simulink model "Estimationdataset1"  (R2023b)
settings: Solver=FixedStepAuto  StartTime=0.0  StopTime=60  FixedStep=1/4096  RelTol=1e-3
(part 1 of 2)
settings Model: Creator=ashle  LastModifiedBy=ashle

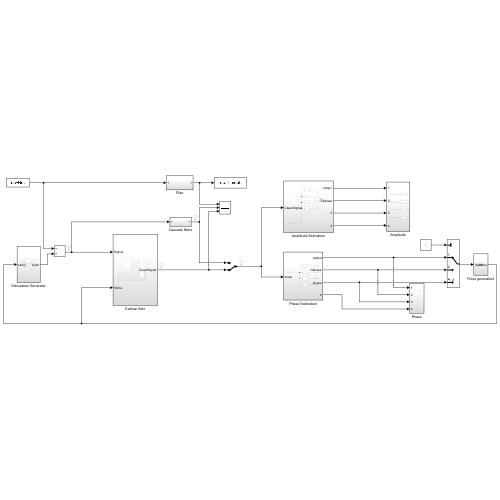
[thumbnail: Simulink's stored preview of the top-level diagram]
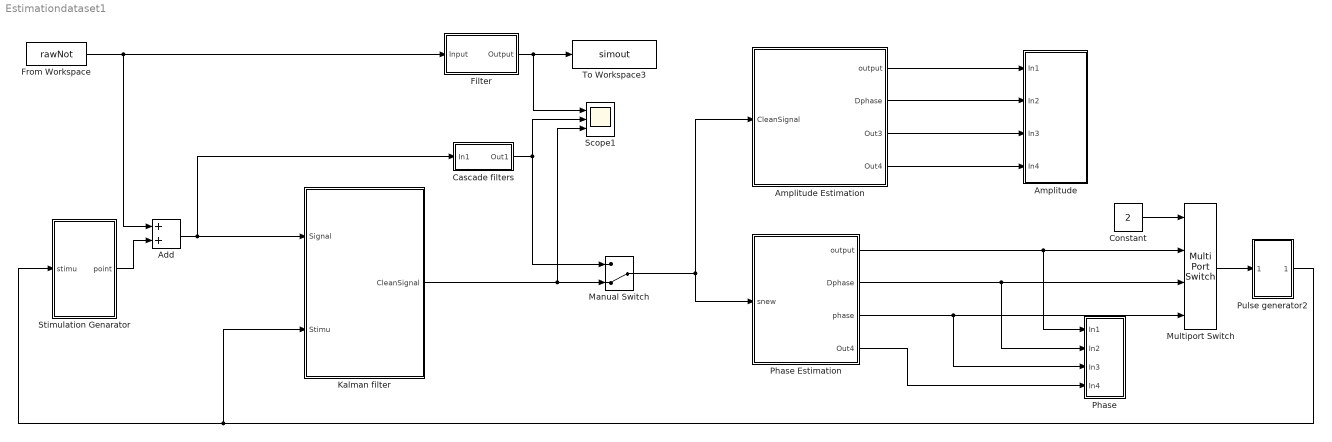
== system Estimationdataset1 ==
  Add : Sum
  Amplitude : Subsystem
  Amplitude Estimation : Subsystem
  Cascade filters : Subsystem
  Constant : Constant  Value=2
  Filter : Subsystem  Tag=FilterWizardSubSystem
      settings: ErrorFcn=dspFilterRealizedInBasicElemsAlgLoopErrFcnCallback
  From Workspace : FromWorkspace  VariableName=rawNot  SampleTime=1/4096
  Kalman filter : Subsystem
  Manual Switch : ManualSwitch  CurrentSetting=0
  Multiport Switch : MultiPortSwitch  SaturateOnIntegerOverflow=off  InputSameDT=off
  Phase : Subsystem
  Phase Estimation : Subsystem
  Pulse generator2 : Subsystem
  Scope1 : Scope  NumInputPorts=3
  Stimulation Genarator : Subsystem
  To Workspace3 : ToWorkspace  VariableName=simout  SampleTime=-1
      settings: Save2DSignal=2-D array (concatenate along first dimension)
  wires:
  Add/1 -> Cascade filters/1(In1), Kalman filter/1(Signal)
  From Workspace/1 -> Filter/1(Input), Add/1
  Stimulation Genarator/1(point) -> Add/2
  Constant/1 -> Multiport Switch/1
  Cascade filters/1(Out1) -> Scope1/2, Manual Switch/1
  Filter/1(Output) -> Scope1/1, To Workspace3/1
  Multiport Switch/1 -> Pulse generator2/1(input)
  Pulse generator2/1(Stimu) -> Stimulation Genarator/1(stimu), Kalman filter/2(Stimu)
  Manual Switch/1 -> Phase Estimation/1(snew), Amplitude Estimation/1(CleanSignal)
  Amplitude Estimation/1(output) -> Amplitude/1(In1)
  Amplitude Estimation/2(Dphase) -> Amplitude/2(In2)
  Amplitude Estimation/3(Out3) -> Amplitude/3(In3)
  Amplitude Estimation/4(Out4) -> Amplitude/4(In4)
  Phase Estimation/1(output) -> Phase/1(In1), Multiport Switch/2
  Phase Estimation/2(Dphase) -> Phase/2(In2), Multiport Switch/3
  Phase Estimation/3(phase) -> Phase/3(In3), Multiport Switch/4
  Phase Estimation/4(Out4) -> Phase/4(In4)
  Kalman filter/1(CleanSignal) -> Scope1/3, Manual Switch/2

== system Estimationdataset1/Amplitude ==
  In1 : Inport
  In2 : Inport  Port=2
  In3 : Inport  Port=3
  In4 : Inport  Port=4
  MW : ToWorkspace  VariableName=simout7  SampleTime=-1
      settings: Save2DSignal=2-D array (concatenate along first dimension)
  NRO : ToWorkspace  VariableName=simout5  SampleTime=-1
      settings: Save2DSignal=2-D array (concatenate along first dimension)
  SS : ToWorkspace  VariableName=simout8  SampleTime=-1
      settings: Save2DSignal=2-D array (concatenate along first dimension)
  ecHT : ToWorkspace  VariableName=simout6  SampleTime=-1
      settings: Save2DSignal=2-D array (concatenate along first dimension)
  wires:
  In2/1 -> NRO/1
  In4/1 -> SS/1
  In1/1 -> ecHT/1
  In3/1 -> MW/1

== system Estimationdataset1/Amplitude Estimation ==
  CleanSignal : Inport
  Hilbert+AR1 : Subsystem
  Moving window : Subsystem
  Non-Resonant Filter1 : Subsystem
  State Space1 : Subsystem
  output : Outport
  Dphase : Outport  Port=2
  Out3 : Outport  Port=3
  Out4 : Outport  Port=4
  wires:
  CleanSignal/1 -> Non-Resonant Filter1/1(snew), Hilbert+AR1/1(input), Moving window/1(input), State Space1/1(CleanSignal)
  Hilbert+AR1/1(output) -> output/1
  Moving window/1(Out1) -> Out3/1
  Non-Resonant Filter1/1(Dphase) -> Dphase/1
  State Space1/1(Out2) -> Out4/1

== system Estimationdataset1/Cascade filters ==
  In1 : Inport
  Filter : Subsystem  Tag=FilterWizardSubSystem
      settings: ErrorFcn=dspFilterRealizedInBasicElemsAlgLoopErrFcnCallback
  Filter1 : Subsystem  Tag=FilterWizardSubSystem
      settings: ErrorFcn=dspFilterRealizedInBasicElemsAlgLoopErrFcnCallback
  Filter2 : Subsystem  Tag=FilterWizardSubSystem
      settings: ErrorFcn=dspFilterRealizedInBasicElemsAlgLoopErrFcnCallback
  Out1 : Outport
  wires:
  In1/1 -> Filter/1(Input)
  Filter/1(Output) -> Filter1/1(Input)
  Filter1/1(Output) -> Filter2/1(Input)
  Filter2/1(Output) -> Out1/1

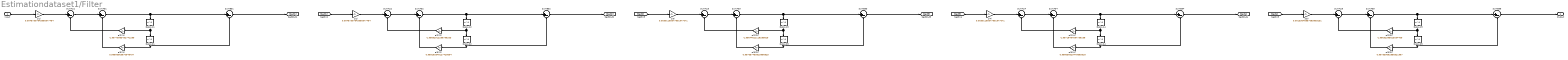
== system Estimationdataset1/Filter ==
  Input : Inport
  Delay{11..15,21..25} (10 alike) : Delay  DelayLength=1  InitialCondition=0
  SumA{21..25,31..35} (10 alike) : Sum  Inputs=|+-  RndMeth=Nearest  SaturateOnIntegerOverflow=on  OutDataTypeStr=Inherit: Same as first input
  SumB{31..35} (5 alike) : Sum  Inputs=|+-  RndMeth=Nearest  SaturateOnIntegerOverflow=on  OutDataTypeStr=Inherit: Same as first input
  a(2)(1) : Gain  Gain=-1.99770983432741289  ParamDataTypeStr=double  RndMeth=Nearest  SaturateOnIntegerOverflow=on  OutDataTypeStr=Inherit: Same as input
  a(2)(2) : Gain  Gain=-1.99852912286796203  ParamDataTypeStr=double  RndMeth=Nearest  SaturateOnIntegerOverflow=on  OutDataTypeStr=Inherit: Same as input
  a(2)(3) : Gain  Gain=-1.99644621118280829  ParamDataTypeStr=double  RndMeth=Nearest  SaturateOnIntegerOverflow=on  OutDataTypeStr=Inherit: Same as input
  a(2)(4) : Gain  Gain=-1.99718487687736168  ParamDataTypeStr=double  RndMeth=Nearest  SaturateOnIntegerOverflow=on  OutDataTypeStr=Inherit: Same as input
  a(2)(5) : Gain  Gain=-1.99632395623034409  ParamDataTypeStr=double  RndMeth=Nearest  SaturateOnIntegerOverflow=on  OutDataTypeStr=Inherit: Same as input
  a(3)(1) : Gain  Gain=0.99906063670948797  ParamDataTypeStr=double  RndMeth=Nearest  SaturateOnIntegerOverflow=on  OutDataTypeStr=Inherit: Same as input
  a(3)(2) : Gain  Gain=0.999293348127428094  ParamDataTypeStr=double  RndMeth=Nearest  SaturateOnIntegerOverflow=on  OutDataTypeStr=Inherit: Same as input
  a(3)(3) : Gain  Gain=0.997657459515996825  ParamDataTypeStr=double  RndMeth=Nearest  SaturateOnIntegerOverflow=on  OutDataTypeStr=Inherit: Same as input
  a(3)(4) : Gain  Gain=0.998036029478669318  ParamDataTypeStr=double  RndMeth=Nearest  SaturateOnIntegerOverflow=on  OutDataTypeStr=Inherit: Same as input
  a(3)(5) : Gain  Gain=0.997339062858321967  ParamDataTypeStr=double  RndMeth=Nearest  SaturateOnIntegerOverflow=on  OutDataTypeStr=Inherit: Same as input
  s(1) : Gain  Gain=0.00457307843590577454  ParamDataTypeStr=double  RndMeth=Nearest  SaturateOnIntegerOverflow=on  OutDataTypeStr=Inherit: Same as input
  s(2) : Gain  Gain=0.00457307843590577454  ParamDataTypeStr=double  RndMeth=Nearest  SaturateOnIntegerOverflow=on  OutDataTypeStr=Inherit: Same as input
  s(3) : Gain  Gain=0.00301199377801977071  ParamDataTypeStr=double  RndMeth=Nearest  SaturateOnIntegerOverflow=on  OutDataTypeStr=Inherit: Same as input
  s(4) : Gain  Gain=0.00301199377801977071  ParamDataTypeStr=double  RndMeth=Nearest  SaturateOnIntegerOverflow=on  OutDataTypeStr=Inherit: Same as input
  s(5) : Gain  Gain=0.00133046857083903231  ParamDataTypeStr=double  RndMeth=Nearest  SaturateOnIntegerOverflow=on  OutDataTypeStr=Inherit: Same as input
  Output : Outport
  wires:
  Input/1 -> s(1)/1
  s(1)/1 -> SumA21/1
  SumA21/1 -> SumA31/1
  SumA31/1 -> SumB31/1, Delay11/1
  SumB31/1 -> [Sect1]
  a(2)(1)/1 -> SumA21/2
  Delay11/1 -> a(2)(1)/1, Delay21/1
  a(3)(1)/1 -> SumA31/2
  Delay21/1 -> a(3)(1)/1, SumB31/2
  [Sect1] -> s(2)/1
  s(2)/1 -> SumA22/1
  SumA22/1 -> SumA32/1
  SumA32/1 -> SumB32/1, Delay12/1
  SumB32/1 -> [Sect2]
  a(2)(2)/1 -> SumA22/2
  Delay12/1 -> a(2)(2)/1, Delay22/1
  a(3)(2)/1 -> SumA32/2
  Delay22/1 -> a(3)(2)/1, SumB32/2
  [Sect2] -> s(3)/1
  s(3)/1 -> SumA23/1
  SumA23/1 -> SumA33/1
  SumA33/1 -> SumB33/1, Delay13/1
  SumB33/1 -> [Sect3]
  a(2)(3)/1 -> SumA23/2
  Delay13/1 -> a(2)(3)/1, Delay23/1
  a(3)(3)/1 -> SumA33/2
  Delay23/1 -> a(3)(3)/1, SumB33/2
  [Sect3] -> s(4)/1
  s(4)/1 -> SumA24/1
  SumA24/1 -> SumA34/1
  SumA34/1 -> SumB34/1, Delay14/1
  SumB34/1 -> [Sect4]
  a(2)(4)/1 -> SumA24/2
  Delay14/1 -> a(2)(4)/1, Delay24/1
  a(3)(4)/1 -> SumA34/2
  Delay24/1 -> a(3)(4)/1, SumB34/2
  [Sect4] -> s(5)/1
  s(5)/1 -> SumA25/1
  SumA25/1 -> SumA35/1
  SumA35/1 -> SumB35/1, Delay15/1
  SumB35/1 -> Output/1
  a(2)(5)/1 -> SumA25/2
  Delay15/1 -> a(2)(5)/1, Delay25/1
  a(3)(5)/1 -> SumA35/2
  Delay25/1 -> a(3)(5)/1, SumB35/2

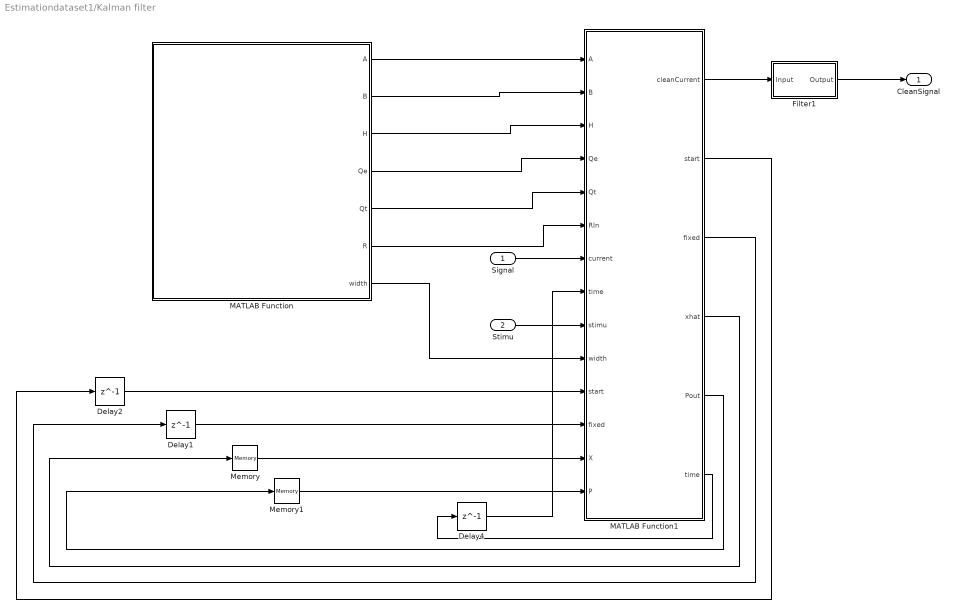
== system Estimationdataset1/Kalman filter ==
  Signal : Inport
  Stimu : Inport  Port=2
  Delay1 : Delay  DelayLength=1  InitialCondition=0
  Delay2 : Delay  DelayLength=1  InitialCondition=0
  Delay4 : Delay  DelayLength=1  InitialCondition=0
  Filter1 : Subsystem  Tag=FilterWizardSubSystem
      settings: ErrorFcn=dspFilterRealizedInBasicElemsAlgLoopErrFcnCallback
  MATLAB Function : MATLAB Function  TreatAsAtomicUnit=on
  MATLAB Function1 : MATLAB Function  TreatAsAtomicUnit=on
  Memory : Memory  InheritSampleTime=on
  Memory1 : Memory  InheritSampleTime=on
  CleanSignal : Outport
  wires:
  Stimu/1 -> MATLAB Function1/9(stimu)
  Memory1/1 -> MATLAB Function1/14(P)
  MATLAB Function1/3(fixed) -> Delay1/1
  Delay1/1 -> MATLAB Function1/12("fixed ")
  MATLAB Function1/2(start) -> Delay2/1
  Delay2/1 -> MATLAB Function1/11("start ")
  Memory/1 -> MATLAB Function1/13(X)
  MATLAB Function1/4(xhat) -> Memory/1
  MATLAB Function1/5(Pout) -> Memory1/1
  MATLAB Function/1(A) -> MATLAB Function1/1(A)
  MATLAB Function/2(B) -> MATLAB Function1/2(B)
  MATLAB Function/3(H) -> MATLAB Function1/3(H)
  MATLAB Function/4(Qe) -> MATLAB Function1/4(Qe)
  MATLAB Function/5(Qt) -> MATLAB Function1/5(Qt)
  MATLAB Function/6(R) -> MATLAB Function1/6(RIn)
  MATLAB Function1/1(cleanCurrent) -> Filter1/1(Input)
  MATLAB Function/7(width) -> MATLAB Function1/10(width)
  Signal/1 -> MATLAB Function1/7(current)
  MATLAB Function1/6(time) -> Delay4/1
  Delay4/1 -> MATLAB Function1/8("time ")
  Filter1/1(Output) -> CleanSignal/1

== system Estimationdataset1/Phase ==
  In1 : Inport
  In2 : Inport  Port=2
  In3 : Inport  Port=3
  In4 : Inport  Port=4
  Scope3 : Scope
  To Workspace : ToWorkspace  VariableName=simout2  SampleTime=-1
      settings: Save2DSignal=2-D array (concatenate along first dimension)
  To Workspace1 : ToWorkspace  VariableName=simout1  SampleTime=-1
      settings: Save2DSignal=2-D array (concatenate along first dimension)
  To Workspace2 : ToWorkspace  VariableName=simout3  SampleTime=-1
      settings: Save2DSignal=2-D array (concatenate along first dimension)
  To Workspace4 : ToWorkspace  VariableName=simout4  SampleTime=-1
      settings: Save2DSignal=2-D array (concatenate along first dimension)
  wires:
  In1/1 -> To Workspace1/1
  In4/1 -> To Workspace4/1
  In3/1 -> To Workspace2/1
  In2/1 -> Scope3/1, To Workspace/1

== system Estimationdataset1/Phase Estimation ==
  snew : Inport
  Hilbert+AR : Subsystem
  Non-Resonant Filter : Subsystem
  State Space : Subsystem
  Zero-crossing : Subsystem
  output : Outport
  Dphase : Outport  Port=2
  phase : Outport  Port=3
  Out4 : Outport  Port=4
  wires:
  Non-Resonant Filter/1(Dphase) -> Dphase/1
  Hilbert+AR/1(output) -> output/1
  Zero-crossing/1(phase) -> phase/1
  snew/1 -> Hilbert+AR/1(input), Non-Resonant Filter/1(snew), State Space/1(CleanSignal), Zero-crossing/1(input)
  State Space/1(Out2) -> Out4/1

== system Estimationdataset1/Pulse generator2 ==
  input : Inport
  Delay5 : Delay  DelayLength=1  InitialCondition=0
  MATLAB Function1 : MATLAB Function  TreatAsAtomicUnit=on
  Stimu : Outport
  wires:
  MATLAB Function1/1(out) -> Delay5/1
  Delay5/1 -> MATLAB Function1/2(previous), Stimu/1
  input/1 -> MATLAB Function1/1(input)

== system Estimationdataset1/Stimulation Genarator ==
  stimu : Inport
  Delay4 : Delay  DelayLength=1  InitialCondition=1
  Enabled Subsystem : Subsystem  TreatAsAtomicUnit=on
  MATLAB Function : MATLAB Function  TreatAsAtomicUnit=on
  Memory : Memory  InheritSampleTime=on  LinearizeAsDelay=on
  point : Outport
  wires:
  MATLAB Function/2(index) -> Delay4/1
  Delay4/1 -> MATLAB Function/3("index ")
  Memory/1 -> MATLAB Function/1(stimulation)
  Enabled Subsystem/1(Out1) -> Memory/1
  MATLAB Function/1(point) -> point/1
  stimu/1 -> Enabled Subsystem/Enable, MATLAB Function/2(stimu)

== system Estimationdataset1/Amplitude Estimation/Hilbert+AR1 ==
  input : Inport
  Buffer : Buffer  N=500  V=499  OutputFrames=off
  Hilbert+AR : MATLAB Function  TreatAsAtomicUnit=on
  output : Outport
  wires:
  Hilbert+AR/1(amp) -> output/1
  input/1 -> Buffer/1
  Buffer/1 -> Hilbert+AR/1(input)

== system Estimationdataset1/Amplitude Estimation/Moving window ==
  input : Inport
  Buffer : Buffer  N=800  V=799  OutputFrames=off
  MATLAB Function : MATLAB Function  TreatAsAtomicUnit=on
  Out1 : Outport
  wires:
  input/1 -> Buffer/1
  Buffer/1 -> MATLAB Function/1(input)
  MATLAB Function/1(amp) -> Out1/1

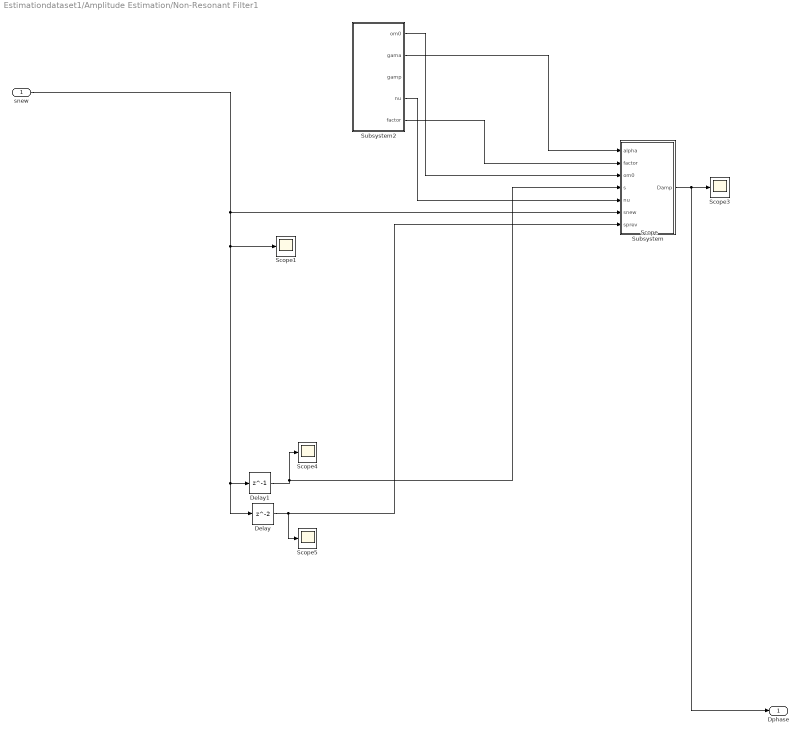
== system Estimationdataset1/Amplitude Estimation/Non-Resonant Filter1 ==
  snew : Inport
  Delay : Delay  InitialCondition=0
  Delay1 : Delay  DelayLength=1  InitialCondition=0
  Scope{,1,3..5} (5 alike) : Scope
  Subsystem : Subsystem
  Subsystem2 : Subsystem
  Dphase : Outport
  wires:
  Delay/1 -> Scope5/1, Subsystem/7(sprev)
  Subsystem2/4(nu) -> Subsystem/5(nu)
  Delay1/1 -> Scope4/1, Subsystem/4(s)
  Subsystem2/1(om0) -> Subsystem/3(om0)
  Subsystem/1(Damp) -> Dphase/1, Scope3/1
  Subsystem2/2(gama) -> Subsystem/1(alpha)
  Subsystem2/5(factor) -> Subsystem/2(factor)
  snew/1 -> Scope1/1, Delay1/1, Delay/1, Subsystem/6(snew)

== system Estimationdataset1/Amplitude Estimation/State Space1 ==
  CleanSignal : Inport
  MATLAB Function2 : MATLAB Function  TreatAsAtomicUnit=on
  MATLAB Function3 : MATLAB Function  TreatAsAtomicUnit=on
  Subsystem : Subsystem
  Out2 : Outport
  wires:
  MATLAB Function2/1(freq) -> MATLAB Function3/1(freq)
  MATLAB Function2/3(ampVec) -> MATLAB Function3/3(ampVector)
  MATLAB Function2/4(sigmaFreqs) -> MATLAB Function3/4(sigmaFreqs)
  MATLAB Function2/2(Fs) -> MATLAB Function3/2(Fs)
  Subsystem/1(Out1) -> Out2/1
  MATLAB Function2/5(sigmaObs) -> Subsystem/1(sigmaObs)
  MATLAB Function3/1(phi) -> Subsystem/2(phi)
  MATLAB Function3/2(Q) -> Subsystem/3(Q)
  MATLAB Function3/3(M) -> Subsystem/4(M)
  CleanSignal/1 -> Subsystem/5(y2)

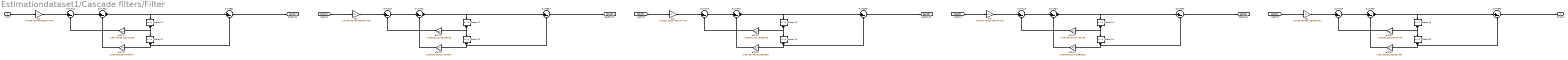
== system Estimationdataset1/Cascade filters/Filter ==
  Input : Inport
  Delay{11..15,21..25} (10 alike) : Delay  DelayLength=1  InitialCondition=0
  SumA{21..25,31..35} (10 alike) : Sum  Inputs=|+-  RndMeth=Nearest  SaturateOnIntegerOverflow=on  OutDataTypeStr=Inherit: Same as first input
  SumB{31..35} (5 alike) : Sum  Inputs=|+-  RndMeth=Nearest  SaturateOnIntegerOverflow=on  OutDataTypeStr=Inherit: Same as first input
  a(2)(1) : Gain  Gain=-1.99770983432741289  ParamDataTypeStr=double  RndMeth=Nearest  SaturateOnIntegerOverflow=on  OutDataTypeStr=Inherit: Same as input
  a(2)(2) : Gain  Gain=-1.99852912286796203  ParamDataTypeStr=double  RndMeth=Nearest  SaturateOnIntegerOverflow=on  OutDataTypeStr=Inherit: Same as input
  a(2)(3) : Gain  Gain=-1.99644621118280829  ParamDataTypeStr=double  RndMeth=Nearest  SaturateOnIntegerOverflow=on  OutDataTypeStr=Inherit: Same as input
  a(2)(4) : Gain  Gain=-1.99718487687736168  ParamDataTypeStr=double  RndMeth=Nearest  SaturateOnIntegerOverflow=on  OutDataTypeStr=Inherit: Same as input
  a(2)(5) : Gain  Gain=-1.99632395623034409  ParamDataTypeStr=double  RndMeth=Nearest  SaturateOnIntegerOverflow=on  OutDataTypeStr=Inherit: Same as input
  a(3)(1) : Gain  Gain=0.99906063670948797  ParamDataTypeStr=double  RndMeth=Nearest  SaturateOnIntegerOverflow=on  OutDataTypeStr=Inherit: Same as input
  a(3)(2) : Gain  Gain=0.999293348127428094  ParamDataTypeStr=double  RndMeth=Nearest  SaturateOnIntegerOverflow=on  OutDataTypeStr=Inherit: Same as input
  a(3)(3) : Gain  Gain=0.997657459515996825  ParamDataTypeStr=double  RndMeth=Nearest  SaturateOnIntegerOverflow=on  OutDataTypeStr=Inherit: Same as input
  a(3)(4) : Gain  Gain=0.998036029478669318  ParamDataTypeStr=double  RndMeth=Nearest  SaturateOnIntegerOverflow=on  OutDataTypeStr=Inherit: Same as input
  a(3)(5) : Gain  Gain=0.997339062858321967  ParamDataTypeStr=double  RndMeth=Nearest  SaturateOnIntegerOverflow=on  OutDataTypeStr=Inherit: Same as input
  s(1) : Gain  Gain=0.00457307843590577454  ParamDataTypeStr=double  RndMeth=Nearest  SaturateOnIntegerOverflow=on  OutDataTypeStr=Inherit: Same as input
  s(2) : Gain  Gain=0.00457307843590577454  ParamDataTypeStr=double  RndMeth=Nearest  SaturateOnIntegerOverflow=on  OutDataTypeStr=Inherit: Same as input
  s(3) : Gain  Gain=0.00301199377801977071  ParamDataTypeStr=double  RndMeth=Nearest  SaturateOnIntegerOverflow=on  OutDataTypeStr=Inherit: Same as input
  s(4) : Gain  Gain=0.00301199377801977071  ParamDataTypeStr=double  RndMeth=Nearest  SaturateOnIntegerOverflow=on  OutDataTypeStr=Inherit: Same as input
  s(5) : Gain  Gain=0.00133046857083903231  ParamDataTypeStr=double  RndMeth=Nearest  SaturateOnIntegerOverflow=on  OutDataTypeStr=Inherit: Same as input
  Output : Outport
  wires:
  Input/1 -> s(1)/1
  s(1)/1 -> SumA21/1
  SumA21/1 -> SumA31/1
  SumA31/1 -> SumB31/1, Delay11/1
  SumB31/1 -> [Sect1]
  a(2)(1)/1 -> SumA21/2
  Delay11/1 -> a(2)(1)/1, Delay21/1
  a(3)(1)/1 -> SumA31/2
  Delay21/1 -> a(3)(1)/1, SumB31/2
  [Sect1] -> s(2)/1
  s(2)/1 -> SumA22/1
  SumA22/1 -> SumA32/1
  SumA32/1 -> SumB32/1, Delay12/1
  SumB32/1 -> [Sect2]
  a(2)(2)/1 -> SumA22/2
  Delay12/1 -> a(2)(2)/1, Delay22/1
  a(3)(2)/1 -> SumA32/2
  Delay22/1 -> a(3)(2)/1, SumB32/2
  [Sect2] -> s(3)/1
  s(3)/1 -> SumA23/1
  SumA23/1 -> SumA33/1
  SumA33/1 -> SumB33/1, Delay13/1
  SumB33/1 -> [Sect3]
  a(2)(3)/1 -> SumA23/2
  Delay13/1 -> a(2)(3)/1, Delay23/1
  a(3)(3)/1 -> SumA33/2
  Delay23/1 -> a(3)(3)/1, SumB33/2
  [Sect3] -> s(4)/1
  s(4)/1 -> SumA24/1
  SumA24/1 -> SumA34/1
  SumA34/1 -> SumB34/1, Delay14/1
  SumB34/1 -> [Sect4]
  a(2)(4)/1 -> SumA24/2
  Delay14/1 -> a(2)(4)/1, Delay24/1
  a(3)(4)/1 -> SumA34/2
  Delay24/1 -> a(3)(4)/1, SumB34/2
  [Sect4] -> s(5)/1
  s(5)/1 -> SumA25/1
  SumA25/1 -> SumA35/1
  SumA35/1 -> SumB35/1, Delay15/1
  SumB35/1 -> Output/1
  a(2)(5)/1 -> SumA25/2
  Delay15/1 -> a(2)(5)/1, Delay25/1
  a(3)(5)/1 -> SumA35/2
  Delay25/1 -> a(3)(5)/1, SumB35/2

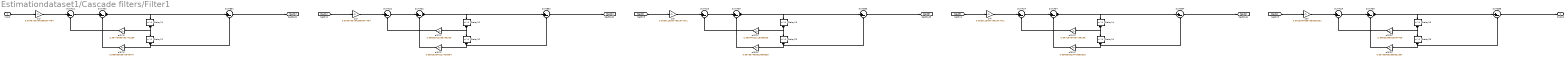
== system Estimationdataset1/Cascade filters/Filter1 ==
  Input : Inport
  Delay{11..15,21..25} (10 alike) : Delay  DelayLength=1  InitialCondition=0
  SumA{21..25,31..35} (10 alike) : Sum  Inputs=|+-  RndMeth=Nearest  SaturateOnIntegerOverflow=on  OutDataTypeStr=Inherit: Same as first input
  SumB{31..35} (5 alike) : Sum  Inputs=|+-  RndMeth=Nearest  SaturateOnIntegerOverflow=on  OutDataTypeStr=Inherit: Same as first input
  a(2)(1) : Gain  Gain=-1.99770983432741289  ParamDataTypeStr=double  RndMeth=Nearest  SaturateOnIntegerOverflow=on  OutDataTypeStr=Inherit: Same as input
  a(2)(2) : Gain  Gain=-1.99852912286796203  ParamDataTypeStr=double  RndMeth=Nearest  SaturateOnIntegerOverflow=on  OutDataTypeStr=Inherit: Same as input
  a(2)(3) : Gain  Gain=-1.99644621118280829  ParamDataTypeStr=double  RndMeth=Nearest  SaturateOnIntegerOverflow=on  OutDataTypeStr=Inherit: Same as input
  a(2)(4) : Gain  Gain=-1.99718487687736168  ParamDataTypeStr=double  RndMeth=Nearest  SaturateOnIntegerOverflow=on  OutDataTypeStr=Inherit: Same as input
  a(2)(5) : Gain  Gain=-1.99632395623034409  ParamDataTypeStr=double  RndMeth=Nearest  SaturateOnIntegerOverflow=on  OutDataTypeStr=Inherit: Same as input
  a(3)(1) : Gain  Gain=0.99906063670948797  ParamDataTypeStr=double  RndMeth=Nearest  SaturateOnIntegerOverflow=on  OutDataTypeStr=Inherit: Same as input
  a(3)(2) : Gain  Gain=0.999293348127428094  ParamDataTypeStr=double  RndMeth=Nearest  SaturateOnIntegerOverflow=on  OutDataTypeStr=Inherit: Same as input
  a(3)(3) : Gain  Gain=0.997657459515996825  ParamDataTypeStr=double  RndMeth=Nearest  SaturateOnIntegerOverflow=on  OutDataTypeStr=Inherit: Same as input
  a(3)(4) : Gain  Gain=0.998036029478669318  ParamDataTypeStr=double  RndMeth=Nearest  SaturateOnIntegerOverflow=on  OutDataTypeStr=Inherit: Same as input
  a(3)(5) : Gain  Gain=0.997339062858321967  ParamDataTypeStr=double  RndMeth=Nearest  SaturateOnIntegerOverflow=on  OutDataTypeStr=Inherit: Same as input
  s(1) : Gain  Gain=0.00457307843590577454  ParamDataTypeStr=double  RndMeth=Nearest  SaturateOnIntegerOverflow=on  OutDataTypeStr=Inherit: Same as input
  s(2) : Gain  Gain=0.00457307843590577454  ParamDataTypeStr=double  RndMeth=Nearest  SaturateOnIntegerOverflow=on  OutDataTypeStr=Inherit: Same as input
  s(3) : Gain  Gain=0.00301199377801977071  ParamDataTypeStr=double  RndMeth=Nearest  SaturateOnIntegerOverflow=on  OutDataTypeStr=Inherit: Same as input
  s(4) : Gain  Gain=0.00301199377801977071  ParamDataTypeStr=double  RndMeth=Nearest  SaturateOnIntegerOverflow=on  OutDataTypeStr=Inherit: Same as input
  s(5) : Gain  Gain=0.00133046857083903231  ParamDataTypeStr=double  RndMeth=Nearest  SaturateOnIntegerOverflow=on  OutDataTypeStr=Inherit: Same as input
  Output : Outport
  wires:
  Input/1 -> s(1)/1
  s(1)/1 -> SumA21/1
  SumA21/1 -> SumA31/1
  SumA31/1 -> SumB31/1, Delay11/1
  SumB31/1 -> [Sect1]
  a(2)(1)/1 -> SumA21/2
  Delay11/1 -> a(2)(1)/1, Delay21/1
  a(3)(1)/1 -> SumA31/2
  Delay21/1 -> a(3)(1)/1, SumB31/2
  [Sect1] -> s(2)/1
  s(2)/1 -> SumA22/1
  SumA22/1 -> SumA32/1
  SumA32/1 -> SumB32/1, Delay12/1
  SumB32/1 -> [Sect2]
  a(2)(2)/1 -> SumA22/2
  Delay12/1 -> a(2)(2)/1, Delay22/1
  a(3)(2)/1 -> SumA32/2
  Delay22/1 -> a(3)(2)/1, SumB32/2
  [Sect2] -> s(3)/1
  s(3)/1 -> SumA23/1
  SumA23/1 -> SumA33/1
  SumA33/1 -> SumB33/1, Delay13/1
  SumB33/1 -> [Sect3]
  a(2)(3)/1 -> SumA23/2
  Delay13/1 -> a(2)(3)/1, Delay23/1
  a(3)(3)/1 -> SumA33/2
  Delay23/1 -> a(3)(3)/1, SumB33/2
  [Sect3] -> s(4)/1
  s(4)/1 -> SumA24/1
  SumA24/1 -> SumA34/1
  SumA34/1 -> SumB34/1, Delay14/1
  SumB34/1 -> [Sect4]
  a(2)(4)/1 -> SumA24/2
  Delay14/1 -> a(2)(4)/1, Delay24/1
  a(3)(4)/1 -> SumA34/2
  Delay24/1 -> a(3)(4)/1, SumB34/2
  [Sect4] -> s(5)/1
  s(5)/1 -> SumA25/1
  SumA25/1 -> SumA35/1
  SumA35/1 -> SumB35/1, Delay15/1
  SumB35/1 -> Output/1
  a(2)(5)/1 -> SumA25/2
  Delay15/1 -> a(2)(5)/1, Delay25/1
  a(3)(5)/1 -> SumA35/2
  Delay25/1 -> a(3)(5)/1, SumB35/2

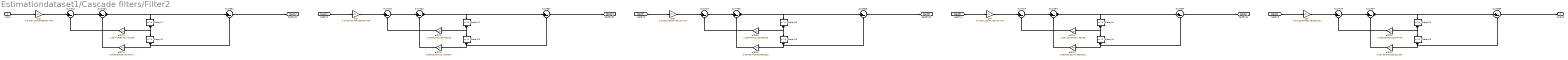
== system Estimationdataset1/Cascade filters/Filter2 ==
  Input : Inport
  Delay{11..15,21..25} (10 alike) : Delay  DelayLength=1  InitialCondition=0
  SumA{21..25,31..35} (10 alike) : Sum  Inputs=|+-  RndMeth=Nearest  SaturateOnIntegerOverflow=on  OutDataTypeStr=Inherit: Same as first input
  SumB{31..35} (5 alike) : Sum  Inputs=|+-  RndMeth=Nearest  SaturateOnIntegerOverflow=on  OutDataTypeStr=Inherit: Same as first input
  a(2)(1) : Gain  Gain=-1.99770983432741289  ParamDataTypeStr=double  RndMeth=Nearest  SaturateOnIntegerOverflow=on  OutDataTypeStr=Inherit: Same as input
  a(2)(2) : Gain  Gain=-1.99852912286796203  ParamDataTypeStr=double  RndMeth=Nearest  SaturateOnIntegerOverflow=on  OutDataTypeStr=Inherit: Same as input
  a(2)(3) : Gain  Gain=-1.99644621118280829  ParamDataTypeStr=double  RndMeth=Nearest  SaturateOnIntegerOverflow=on  OutDataTypeStr=Inherit: Same as input
  a(2)(4) : Gain  Gain=-1.99718487687736168  ParamDataTypeStr=double  RndMeth=Nearest  SaturateOnIntegerOverflow=on  OutDataTypeStr=Inherit: Same as input
  a(2)(5) : Gain  Gain=-1.99632395623034409  ParamDataTypeStr=double  RndMeth=Nearest  SaturateOnIntegerOverflow=on  OutDataTypeStr=Inherit: Same as input
  a(3)(1) : Gain  Gain=0.99906063670948797  ParamDataTypeStr=double  RndMeth=Nearest  SaturateOnIntegerOverflow=on  OutDataTypeStr=Inherit: Same as input
  a(3)(2) : Gain  Gain=0.999293348127428094  ParamDataTypeStr=double  RndMeth=Nearest  SaturateOnIntegerOverflow=on  OutDataTypeStr=Inherit: Same as input
  a(3)(3) : Gain  Gain=0.997657459515996825  ParamDataTypeStr=double  RndMeth=Nearest  SaturateOnIntegerOverflow=on  OutDataTypeStr=Inherit: Same as input
  a(3)(4) : Gain  Gain=0.998036029478669318  ParamDataTypeStr=double  RndMeth=Nearest  SaturateOnIntegerOverflow=on  OutDataTypeStr=Inherit: Same as input
  a(3)(5) : Gain  Gain=0.997339062858321967  ParamDataTypeStr=double  RndMeth=Nearest  SaturateOnIntegerOverflow=on  OutDataTypeStr=Inherit: Same as input
  s(1) : Gain  Gain=0.00457307843590577454  ParamDataTypeStr=double  RndMeth=Nearest  SaturateOnIntegerOverflow=on  OutDataTypeStr=Inherit: Same as input
  s(2) : Gain  Gain=0.00457307843590577454  ParamDataTypeStr=double  RndMeth=Nearest  SaturateOnIntegerOverflow=on  OutDataTypeStr=Inherit: Same as input
  s(3) : Gain  Gain=0.00301199377801977071  ParamDataTypeStr=double  RndMeth=Nearest  SaturateOnIntegerOverflow=on  OutDataTypeStr=Inherit: Same as input
  s(4) : Gain  Gain=0.00301199377801977071  ParamDataTypeStr=double  RndMeth=Nearest  SaturateOnIntegerOverflow=on  OutDataTypeStr=Inherit: Same as input
  s(5) : Gain  Gain=0.00133046857083903231  ParamDataTypeStr=double  RndMeth=Nearest  SaturateOnIntegerOverflow=on  OutDataTypeStr=Inherit: Same as input
  Output : Outport
  wires:
  Input/1 -> s(1)/1
  s(1)/1 -> SumA21/1
  SumA21/1 -> SumA31/1
  SumA31/1 -> SumB31/1, Delay11/1
  SumB31/1 -> [Sect1]
  a(2)(1)/1 -> SumA21/2
  Delay11/1 -> a(2)(1)/1, Delay21/1
  a(3)(1)/1 -> SumA31/2
  Delay21/1 -> a(3)(1)/1, SumB31/2
  [Sect1] -> s(2)/1
  s(2)/1 -> SumA22/1
  SumA22/1 -> SumA32/1
  SumA32/1 -> SumB32/1, Delay12/1
  SumB32/1 -> [Sect2]
  a(2)(2)/1 -> SumA22/2
  Delay12/1 -> a(2)(2)/1, Delay22/1
  a(3)(2)/1 -> SumA32/2
  Delay22/1 -> a(3)(2)/1, SumB32/2
  [Sect2] -> s(3)/1
  s(3)/1 -> SumA23/1
  SumA23/1 -> SumA33/1
  SumA33/1 -> SumB33/1, Delay13/1
  SumB33/1 -> [Sect3]
  a(2)(3)/1 -> SumA23/2
  Delay13/1 -> a(2)(3)/1, Delay23/1
  a(3)(3)/1 -> SumA33/2
  Delay23/1 -> a(3)(3)/1, SumB33/2
  [Sect3] -> s(4)/1
  s(4)/1 -> SumA24/1
  SumA24/1 -> SumA34/1
  SumA34/1 -> SumB34/1, Delay14/1
  SumB34/1 -> [Sect4]
  a(2)(4)/1 -> SumA24/2
  Delay14/1 -> a(2)(4)/1, Delay24/1
  a(3)(4)/1 -> SumA34/2
  Delay24/1 -> a(3)(4)/1, SumB34/2
  [Sect4] -> s(5)/1
  s(5)/1 -> SumA25/1
  SumA25/1 -> SumA35/1
  SumA35/1 -> SumB35/1, Delay15/1
  SumB35/1 -> Output/1
  a(2)(5)/1 -> SumA25/2
  Delay15/1 -> a(2)(5)/1, Delay25/1
  a(3)(5)/1 -> SumA35/2
  Delay25/1 -> a(3)(5)/1, SumB35/2

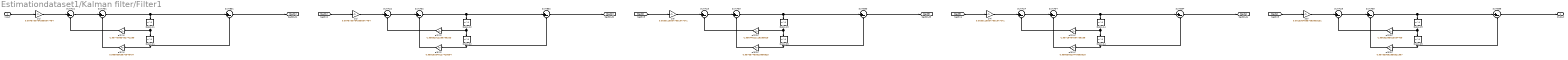
== system Estimationdataset1/Kalman filter/Filter1 ==
  Input : Inport
  Delay{11..15,21..25} (10 alike) : Delay  DelayLength=1  InitialCondition=0
  SumA{21..25,31..35} (10 alike) : Sum  Inputs=|+-  RndMeth=Nearest  SaturateOnIntegerOverflow=on  OutDataTypeStr=Inherit: Same as first input
  SumB{31..35} (5 alike) : Sum  Inputs=|+-  RndMeth=Nearest  SaturateOnIntegerOverflow=on  OutDataTypeStr=Inherit: Same as first input
  a(2)(1) : Gain  Gain=-1.99770983432741289  ParamDataTypeStr=double  RndMeth=Nearest  SaturateOnIntegerOverflow=on  OutDataTypeStr=Inherit: Same as input
  a(2)(2) : Gain  Gain=-1.99852912286796203  ParamDataTypeStr=double  RndMeth=Nearest  SaturateOnIntegerOverflow=on  OutDataTypeStr=Inherit: Same as input
  a(2)(3) : Gain  Gain=-1.99644621118280829  ParamDataTypeStr=double  RndMeth=Nearest  SaturateOnIntegerOverflow=on  OutDataTypeStr=Inherit: Same as input
  a(2)(4) : Gain  Gain=-1.99718487687736168  ParamDataTypeStr=double  RndMeth=Nearest  SaturateOnIntegerOverflow=on  OutDataTypeStr=Inherit: Same as input
  a(2)(5) : Gain  Gain=-1.99632395623034409  ParamDataTypeStr=double  RndMeth=Nearest  SaturateOnIntegerOverflow=on  OutDataTypeStr=Inherit: Same as input
  a(3)(1) : Gain  Gain=0.99906063670948797  ParamDataTypeStr=double  RndMeth=Nearest  SaturateOnIntegerOverflow=on  OutDataTypeStr=Inherit: Same as input
  a(3)(2) : Gain  Gain=0.999293348127428094  ParamDataTypeStr=double  RndMeth=Nearest  SaturateOnIntegerOverflow=on  OutDataTypeStr=Inherit: Same as input
  a(3)(3) : Gain  Gain=0.997657459515996825  ParamDataTypeStr=double  RndMeth=Nearest  SaturateOnIntegerOverflow=on  OutDataTypeStr=Inherit: Same as input
  a(3)(4) : Gain  Gain=0.998036029478669318  ParamDataTypeStr=double  RndMeth=Nearest  SaturateOnIntegerOverflow=on  OutDataTypeStr=Inherit: Same as input
  a(3)(5) : Gain  Gain=0.997339062858321967  ParamDataTypeStr=double  RndMeth=Nearest  SaturateOnIntegerOverflow=on  OutDataTypeStr=Inherit: Same as input
  s(1) : Gain  Gain=0.00457307843590577454  ParamDataTypeStr=double  RndMeth=Nearest  SaturateOnIntegerOverflow=on  OutDataTypeStr=Inherit: Same as input
  s(2) : Gain  Gain=0.00457307843590577454  ParamDataTypeStr=double  RndMeth=Nearest  SaturateOnIntegerOverflow=on  OutDataTypeStr=Inherit: Same as input
  s(3) : Gain  Gain=0.00301199377801977071  ParamDataTypeStr=double  RndMeth=Nearest  SaturateOnIntegerOverflow=on  OutDataTypeStr=Inherit: Same as input
  s(4) : Gain  Gain=0.00301199377801977071  ParamDataTypeStr=double  RndMeth=Nearest  SaturateOnIntegerOverflow=on  OutDataTypeStr=Inherit: Same as input
  s(5) : Gain  Gain=0.00133046857083903231  ParamDataTypeStr=double  RndMeth=Nearest  SaturateOnIntegerOverflow=on  OutDataTypeStr=Inherit: Same as input
  Output : Outport
  wires:
  Input/1 -> s(1)/1
  s(1)/1 -> SumA21/1
  SumA21/1 -> SumA31/1
  SumA31/1 -> SumB31/1, Delay11/1
  SumB31/1 -> [Sect1]
  a(2)(1)/1 -> SumA21/2
  Delay11/1 -> a(2)(1)/1, Delay21/1
  a(3)(1)/1 -> SumA31/2
  Delay21/1 -> a(3)(1)/1, SumB31/2
  [Sect1] -> s(2)/1
  s(2)/1 -> SumA22/1
  SumA22/1 -> SumA32/1
  SumA32/1 -> SumB32/1, Delay12/1
  SumB32/1 -> [Sect2]
  a(2)(2)/1 -> SumA22/2
  Delay12/1 -> a(2)(2)/1, Delay22/1
  a(3)(2)/1 -> SumA32/2
  Delay22/1 -> a(3)(2)/1, SumB32/2
  [Sect2] -> s(3)/1
  s(3)/1 -> SumA23/1
  SumA23/1 -> SumA33/1
  SumA33/1 -> SumB33/1, Delay13/1
  SumB33/1 -> [Sect3]
  a(2)(3)/1 -> SumA23/2
  Delay13/1 -> a(2)(3)/1, Delay23/1
  a(3)(3)/1 -> SumA33/2
  Delay23/1 -> a(3)(3)/1, SumB33/2
  [Sect3] -> s(4)/1
  s(4)/1 -> SumA24/1
  SumA24/1 -> SumA34/1
  SumA34/1 -> SumB34/1, Delay14/1
  SumB34/1 -> [Sect4]
  a(2)(4)/1 -> SumA24/2
  Delay14/1 -> a(2)(4)/1, Delay24/1
  a(3)(4)/1 -> SumA34/2
  Delay24/1 -> a(3)(4)/1, SumB34/2
  [Sect4] -> s(5)/1
  s(5)/1 -> SumA25/1
  SumA25/1 -> SumA35/1
  SumA35/1 -> SumB35/1, Delay15/1
  SumB35/1 -> Output/1
  a(2)(5)/1 -> SumA25/2
  Delay15/1 -> a(2)(5)/1, Delay25/1
  a(3)(5)/1 -> SumA35/2
  Delay25/1 -> a(3)(5)/1, SumB35/2

== system Estimationdataset1/Phase Estimation/Hilbert+AR ==
  input : Inport
  Buffer : Buffer  N=500  V=499  OutputFrames=off
  Hilbert+AR : MATLAB Function  TreatAsAtomicUnit=on
  output : Outport
  wires:
  Hilbert+AR/1(phase) -> output/1
  input/1 -> Buffer/1
  Buffer/1 -> Hilbert+AR/1(input)

== system Estimationdataset1/Phase Estimation/Non-Resonant Filter ==
  snew : Inport
  Delay : Delay  InitialCondition=0
  Delay1 : Delay  DelayLength=1  InitialCondition=0
  Scope{1..2,4..5} (4 alike) : Scope
  Subsystem1 : Subsystem
  Subsystem2 : Subsystem
  Dphase : Outport
  wires:
  Delay/1 -> Scope5/1, Subsystem1/6(sprev)
  Subsystem2/4(nu) -> Subsystem1/4(nu)
  Delay1/1 -> Scope4/1, Subsystem1/3(s)
  Subsystem2/1(om0) -> Subsystem1/2(om0)
  Subsystem2/3(gamp) -> Subsystem1/1(alpha)
  Subsystem1/1(Dphase) -> Dphase/1, Scope2/1
  snew/1 -> Scope1/1, Subsystem1/5(snew), Delay1/1, Delay/1

== system Estimationdataset1/Phase Estimation/State Space ==
  CleanSignal : Inport
  MATLAB Function2 : MATLAB Function  TreatAsAtomicUnit=on
  MATLAB Function3 : MATLAB Function  TreatAsAtomicUnit=on
  Subsystem : Subsystem
  Out2 : Outport
  wires:
  MATLAB Function2/1(freq) -> MATLAB Function3/1(freq)
  MATLAB Function2/3(ampVec) -> MATLAB Function3/3(ampVector)
  MATLAB Function2/4(sigmaFreqs) -> MATLAB Function3/4(sigmaFreqs)
  MATLAB Function2/2(Fs) -> MATLAB Function3/2(Fs)
  Subsystem/1(Out1) -> Out2/1
  MATLAB Function2/5(sigmaObs) -> Subsystem/1(sigmaObs)
  MATLAB Function3/1(phi) -> Subsystem/2(phi)
  MATLAB Function3/2(Q) -> Subsystem/3(Q)
  MATLAB Function3/3(M) -> Subsystem/4(M)
  CleanSignal/1 -> Subsystem/5(y2)

== system Estimationdataset1/Phase Estimation/Zero-crossing ==
  input : Inport
  Delay : Delay  DelayLength=1  InitialCondition=0
  Delay1 : Delay  DelayLength=1  InitialCondition=0
  Delay2 : Delay  DelayLength=1  InitialCondition=0
  Delay3 : Delay  DelayLength=1  InitialCondition=20
  Zero-crossing : MATLAB Function  TreatAsAtomicUnit=on
  phase : Outport
  wires:
  Zero-crossing/2(out) -> Delay/1
  Zero-crossing/1(phase_wrapped) -> phase/1
  Zero-crossing/3(time) -> Delay2/1
  Zero-crossing/4(instantaneous_frequency) -> Delay3/1
  Delay3/1 -> Zero-crossing/5(frequency)
  Delay1/1 -> Zero-crossing/4(last_crossing)
  Delay2/1 -> Zero-crossing/2("time ")
  Delay/1 -> Zero-crossing/3(last)
  Zero-crossing/5(crossing) -> Delay1/1
  input/1 -> Zero-crossing/1(input)

== system Estimationdataset1/Stimulation Genarator/Enabled Subsystem ==
  Enable : EnablePort
  MATLAB Function : MATLAB Function  TreatAsAtomicUnit=on
  Round : Rounding  Operator=round
  Selector : Selector  NumberOfDimensions=2  InputPortWidth=3  IndexOptions=Index vector (dialog),Index vector (port)  Indices=[1:42],[1 42]  OutputSizes=1,1
  Uniform Random Number : UniformRandomNumber  Minimum=0.5  Maximum=25.4  SampleTime=1/4096
  Out1 : Outport
  wires:
  Uniform Random Number/1 -> Round/1
  MATLAB Function/1(Stimulation) -> Selector/1
  Selector/1 -> Out1/1
  Round/1 -> Selector/2

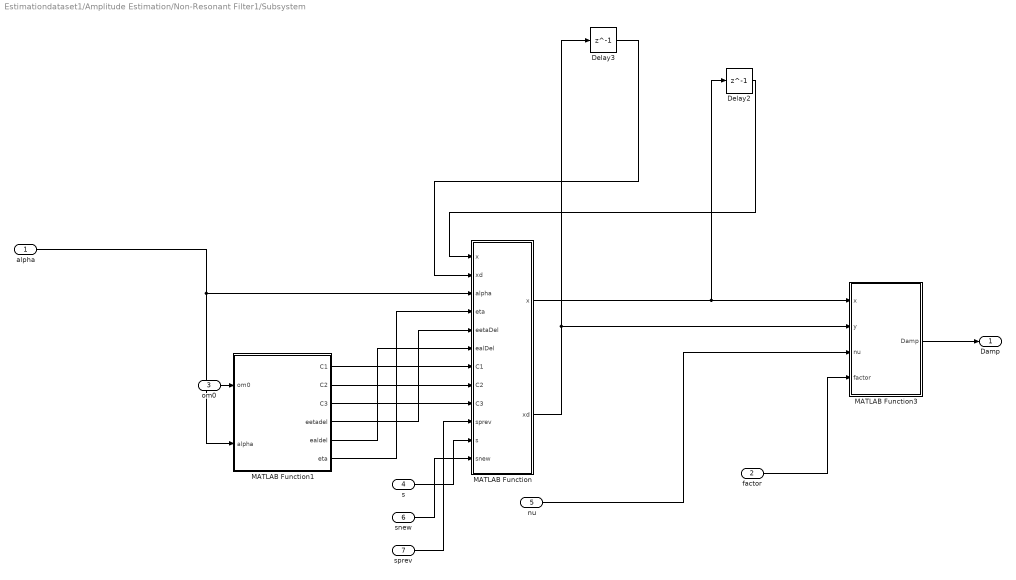
== system Estimationdataset1/Amplitude Estimation/Non-Resonant Filter1/Subsystem ==
  alpha : Inport
  factor : Inport  Port=2
  om0 : Inport  Port=3
  s : Inport  Port=4
  nu : Inport  Port=5
  snew : Inport  Port=6
  sprev : Inport  Port=7
  Delay2 : Delay  DelayLength=1  InitialCondition=0
  Delay3 : Delay  DelayLength=1  InitialCondition=0
  MATLAB Function : MATLAB Function  TreatAsAtomicUnit=on
  MATLAB Function1 : MATLAB Function  TreatAsAtomicUnit=on
  MATLAB Function3 : MATLAB Function  TreatAsAtomicUnit=on
  Damp : Outport
  wires:
  MATLAB Function1/4(eetadel) -> MATLAB Function/5(eetaDel)
  MATLAB Function1/5(ealdel) -> MATLAB Function/6(ealDel)
  MATLAB Function/1(x) -> Delay2/1, MATLAB Function3/1(x)
  MATLAB Function/2(xd) -> Delay3/1, MATLAB Function3/2(y)
  MATLAB Function1/2(C2) -> MATLAB Function/8(C2)
  MATLAB Function1/6(eta) -> MATLAB Function/4(eta)
  MATLAB Function1/3(C3) -> MATLAB Function/9(C3)
  MATLAB Function1/1(C1) -> MATLAB Function/7(C1)
  snew/1 -> MATLAB Function/12(snew)
  alpha/1 -> MATLAB Function1/2(alpha), MATLAB Function/3(alpha)
  nu/1 -> MATLAB Function3/3(nu)
  Delay3/1 -> MATLAB Function/2("xd ")
  Delay2/1 -> MATLAB Function/1("x ")
  MATLAB Function3/1(Damp) -> Damp/1
  factor/1 -> MATLAB Function3/4(factor)
  sprev/1 -> MATLAB Function/10(sprev)
  s/1 -> MATLAB Function/11(s)
  om0/1 -> MATLAB Function1/1(om0)

== system Estimationdataset1/Amplitude Estimation/Non-Resonant Filter1/Subsystem2 ==
  MATLAB Function2 : MATLAB Function  TreatAsAtomicUnit=on
  om0 : Outport
  gama : Outport  Port=2
  gamp : Outport  Port=3
  nu : Outport  Port=4
  factor : Outport  Port=5
  wires:
  MATLAB Function2/4(nu) -> nu/1
  MATLAB Function2/2(gama) -> gama/1
  MATLAB Function2/1(om0) -> om0/1
  MATLAB Function2/5(factor) -> factor/1
  MATLAB Function2/3(gamp) -> gamp/1

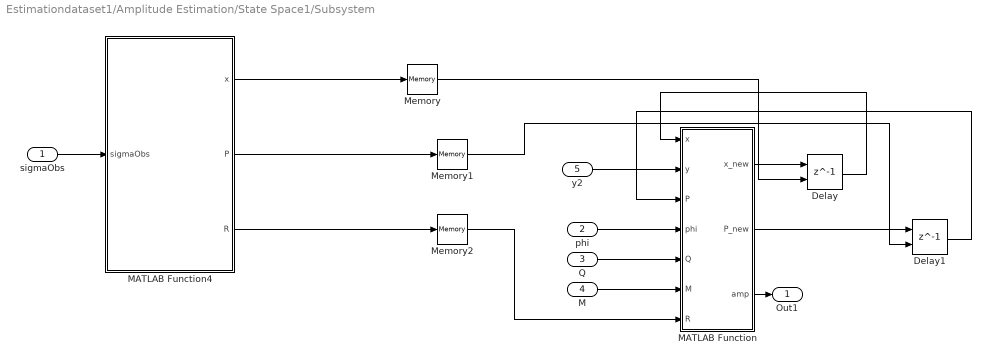
== system Estimationdataset1/Amplitude Estimation/State Space1/Subsystem ==
  sigmaObs : Inport
  phi : Inport  Port=2
  Q : Inport  Port=3
  M : Inport  Port=4
  y2 : Inport  Port=5
  Delay : Delay  DelayLength=1  InitialConditionSource=Input port  InitialCondition=0
      settings: InputPortMap=u0,p4
  Delay1 : Delay  DelayLength=1  InitialConditionSource=Input port  InitialCondition=0
      settings: InputPortMap=u0,p4
  MATLAB Function : MATLAB Function  TreatAsAtomicUnit=on
  MATLAB Function4 : MATLAB Function  TreatAsAtomicUnit=on
  Memory : Memory
  Memory1 : Memory
  Memory2 : Memory
  Out1 : Outport
  wires:
  MATLAB Function4/1(x) -> Memory/1
  MATLAB Function4/2(P) -> Memory1/1
  sigmaObs/1 -> MATLAB Function4/1(sigmaObs)
  MATLAB Function4/3(R) -> Memory2/1
  Delay/1 -> MATLAB Function/1(x)
  MATLAB Function/1(x_new) -> Delay/1
  MATLAB Function/3(amp) -> Out1/1
  M/1 -> MATLAB Function/6(M)
  Memory1/1 -> Delay1/2
  Delay1/1 -> MATLAB Function/3(P)
  Q/1 -> MATLAB Function/5(Q)
  Memory2/1 -> MATLAB Function/7(R)
  MATLAB Function/2(P_new) -> Delay1/1
  phi/1 -> MATLAB Function/4(phi)
  y2/1 -> MATLAB Function/2(y)
  Memory/1 -> Delay/2

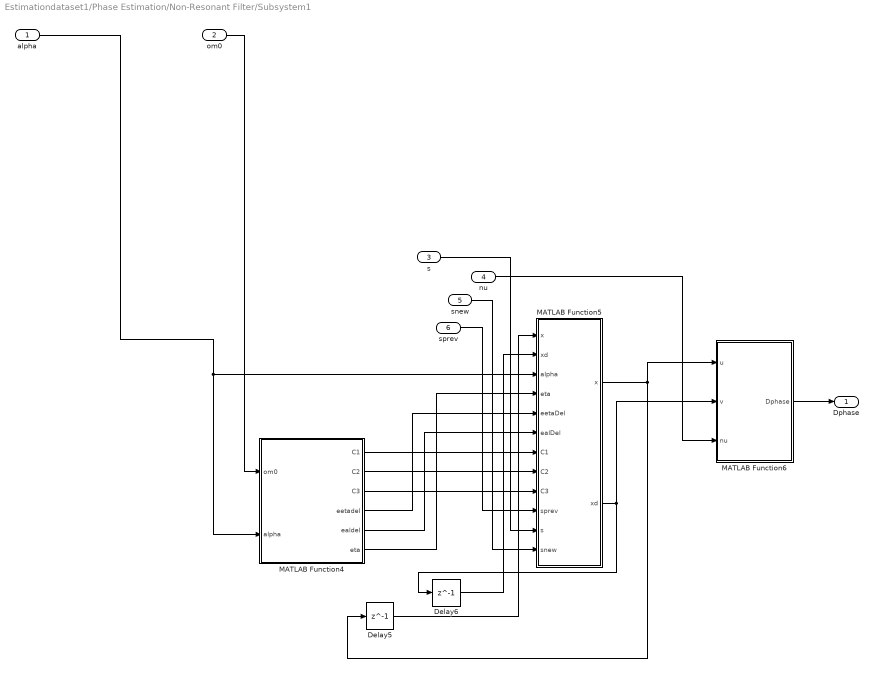
== system Estimationdataset1/Phase Estimation/Non-Resonant Filter/Subsystem1 ==
  alpha : Inport
  om0 : Inport  Port=2
  s : Inport  Port=3
  nu : Inport  Port=4
  snew : Inport  Port=5
  sprev : Inport  Port=6
  Delay5 : Delay  DelayLength=1  InitialCondition=0
  Delay6 : Delay  DelayLength=1  InitialCondition=0
  MATLAB Function4 : MATLAB Function  TreatAsAtomicUnit=on
  MATLAB Function5 : MATLAB Function  TreatAsAtomicUnit=on
  MATLAB Function6 : MATLAB Function  TreatAsAtomicUnit=on
  Dphase : Outport
  wires:
  MATLAB Function4/3(C3) -> MATLAB Function5/9(C3)
  Delay6/1 -> MATLAB Function5/2("xd ")
  alpha/1 -> MATLAB Function4/2(alpha), MATLAB Function5/3(alpha)
  MATLAB Function5/2(xd) -> MATLAB Function6/2(v), Delay6/1
  MATLAB Function4/2(C2) -> MATLAB Function5/8(C2)
  MATLAB Function5/1(x) -> MATLAB Function6/1(u), Delay5/1
  MATLAB Function4/4(eetadel) -> MATLAB Function5/5(eetaDel)
  MATLAB Function4/5(ealdel) -> MATLAB Function5/6(ealDel)
  MATLAB Function4/6(eta) -> MATLAB Function5/4(eta)
  MATLAB Function4/1(C1) -> MATLAB Function5/7(C1)
  Delay5/1 -> MATLAB Function5/1("x ")
  MATLAB Function6/1(Dphase) -> Dphase/1
  om0/1 -> MATLAB Function4/1(om0)
  nu/1 -> MATLAB Function6/3(nu)
  snew/1 -> MATLAB Function5/12(snew)
  s/1 -> MATLAB Function5/11(s)
  sprev/1 -> MATLAB Function5/10(sprev)

== system Estimationdataset1/Phase Estimation/Non-Resonant Filter/Subsystem2 ==
  MATLAB Function2 : MATLAB Function  TreatAsAtomicUnit=on
  om0 : Outport
  gama : Outport  Port=2
  gamp : Outport  Port=3
  nu : Outport  Port=4
  factor : Outport  Port=5
  wires:
  MATLAB Function2/4(nu) -> nu/1
  MATLAB Function2/2(gama) -> gama/1
  MATLAB Function2/1(om0) -> om0/1
  MATLAB Function2/5(factor) -> factor/1
  MATLAB Function2/3(gamp) -> gamp/1

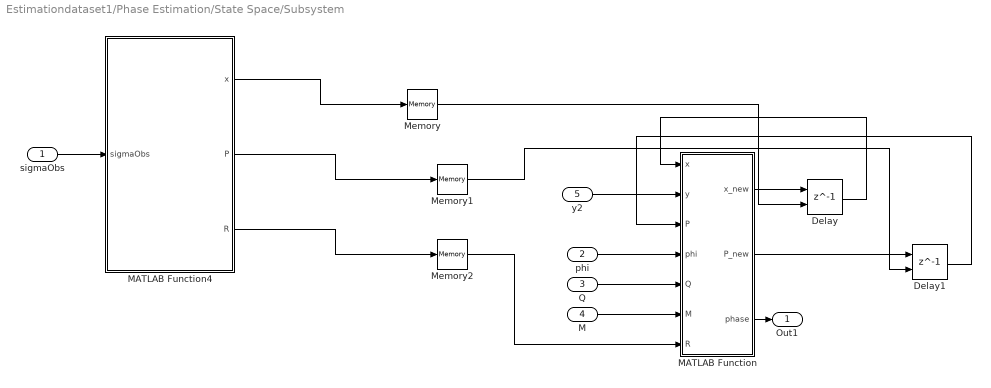
== system Estimationdataset1/Phase Estimation/State Space/Subsystem ==
  sigmaObs : Inport
  phi : Inport  Port=2
  Q : Inport  Port=3
  M : Inport  Port=4
  y2 : Inport  Port=5
  Delay : Delay  DelayLength=1  InitialConditionSource=Input port  InitialCondition=0
      settings: InputPortMap=u0,p4
  Delay1 : Delay  DelayLength=1  InitialConditionSource=Input port  InitialCondition=0
      settings: InputPortMap=u0,p4
  MATLAB Function : MATLAB Function  TreatAsAtomicUnit=on
  MATLAB Function4 : MATLAB Function  TreatAsAtomicUnit=on
  Memory : Memory
  Memory1 : Memory
  Memory2 : Memory
  Out1 : Outport
  wires:
  MATLAB Function4/1(x) -> Memory/1
  MATLAB Function4/2(P) -> Memory1/1
  sigmaObs/1 -> MATLAB Function4/1(sigmaObs)
  MATLAB Function4/3(R) -> Memory2/1
  Delay/1 -> MATLAB Function/1(x)
  MATLAB Function/1(x_new) -> Delay/1
  MATLAB Function/3(phase) -> Out1/1
  M/1 -> MATLAB Function/6(M)
  Memory1/1 -> Delay1/2
  Delay1/1 -> MATLAB Function/3(P)
  Q/1 -> MATLAB Function/5(Q)
  Memory2/1 -> MATLAB Function/7(R)
  MATLAB Function/2(P_new) -> Delay1/1
  phi/1 -> MATLAB Function/4(phi)
  y2/1 -> MATLAB Function/2(y)
  Memory/1 -> Delay/2

== matlab function Estimationdataset1/Kalman filter/MATLAB Function1 ==
  data: A input; B input; H input; Qe input; Qt input; RIn input; current input; time input; cleanCurrent output; stimu input; width input; start input; fixed input; X input; P input; start output; fixed output; xhat output; Pout output; time output
function [cleanCurrent, start, fixed,xhat,Pout,time]   = KalmanFilter(A,B,H,Qe,Qt,RIn,current,time,stimu,width,start,fixed,X,P)
if isempty(start)
    start = 0;
end
if isempty(fixed)
    fixed = 0;
end
if isempty(P)
    P = [1 0;0 1];
end
if isempty(X)
    X = [0 0;0 0];
end
if isempty(time)
    time = 1;
end

% Sure stimulation duration tpeaks~fixed
if stimu == 1
        start = time;
        fixed = time + width;
end


if time > start && time < fixed
        % During artifact
        % Set noise matrices to high values so only model is trusted
        Q = Qt;
        R = RIn;
        u = 0;
else
        % During artifact-free sections
        Q = Qe;
        R = 0;
        u = 0;
end

% Kalman filtering
x_time = A * X + B * u;
P_time = A * P * A' + Q;

K = P_time * H' * pinv(H * P_time * H' + R);
epsilon = current - H * x_time;

xhat = x_time + K .* epsilon;
% Output signal
cleanCurrent = xhat(1,1);

Pout = P_time - K * H * P_time;
time = time+1;

end
